simulink model "PathFollowComp"  (R2015a)
settings: Solver=ode3  StartTime=0.0  StopTime=400  FixedStep=0.01  RelTol=1e-3
values from neighbouring files (symbols this model uses):
  K_eta = 1    [CD.m]    (also in PathFollowCompScript.m = 0.21)
  lambda_0 = atan2(lambda_vec_0(2),lambda_vec_0(1))    [CD.m]    (also in PathFollowCompScript.m)
  rangethresh = 50    [PathFollowCompScript.m]
undefined symbols (not defined in the file): Initial_Heading, Initial_Position, Initial_Position_O
libraries: simulink x13, aerolibtransform2 x4
(part 2 of 2)

== matlab function PathFollowComp/Eta1/wrap1 ==
  data: u input; y output
function y = fcn(u)
%#codegen

%u2 = mod(u,2*pi);
u2 = u - 2*pi*floor( (u+pi)/(2*pi) ); 
y = u2;

== matlab function PathFollowComp/Lambda1/atan2_unwrap/MATLAB Function1 ==
  data: u input; y output; upast input; bias input; bias1 output
function [y, bias1] = fcn(u,upast,bias)
newbias = 0;
if u-upast > 3*pi/2
    newbias = -4*pi/2;
end
if u-upast < -3*pi/2
   newbias = +4*pi/2;
end
bias1 = bias + newbias;
y = u+bias1;
